simulink model "Subsystem"  (R2020a)
settings: Solver=VariableStepAuto  StartTime=0.0  StopTime=10.0  RelTol=1e-3
model workspace (MAT data in the model file):
  Ki = Simulink.Parameter
  Ki.Value = 50
  Ki.DataType = 'auto'
  Ki.Dimensions = [1 1]
  Kp = Simulink.Parameter
  Kp.Value = 800
  Kp.DataType = 'auto'
  Kp.Dimensions = [1 1]
  ki = Simulink.Parameter
  ki.Value = 50
  ki.DataType = 'auto'
  ki.Dimensions = [1 1]
  kp = Simulink.Parameter
  kp.Value = 800
  kp.DataType = 'auto'
  kp.Dimensions = [1 1]
undefined symbols (not defined in the file): b, m
settings Model: Creator=Riyansh  LastModifiedBy=Riyansh
settings DataIOCC: SaveOutput=off  SaveTime=off

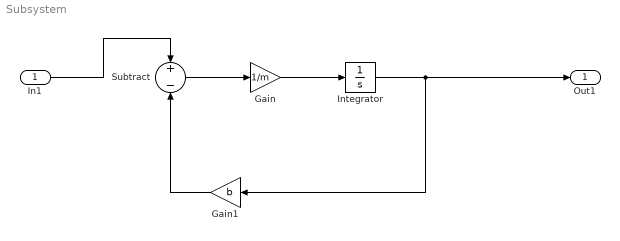
== system Subsystem ==
  In1 : Inport  OutDataTypeStr=double  PortDimensions=1  SampleTime=0
  "Gain " : Gain  Gain=1/m
  "Gain1 " : Gain  Gain=b
  "Integrator " : Integrator
  Subtract : Sum  Inputs=+-
  Out1 : Outport  OutDataTypeStr=double  PortDimensions=1  SampleTime=0
  wires:
  "Gain "/1 -> "Integrator "/1
  In1/1 -> Subtract/1
  "Gain1 "/1 -> Subtract/2
  Subtract/1 -> "Gain "/1
  "Integrator "/1 -> "Gain1 "/1, Out1/1
